simulink model "KF_R_estimation"  (R2021b)
settings: Solver=FixedStepAuto  StartTime=0.0  StopTime=20  MaxStep=1  MinStep=1e-3  RelTol=1e-3
values from neighbouring files (symbols this model uses):
  delta_t = 1/fs    (= 0.001)    [Extended_kalman_filter.m]    (also in kalman_filter.m)
  fs = 1000    [Extended_kalman_filter.m]    (also in kalman_filter.m)
  H = [0,1,1,0,0,0 ... (first row only)    [Extended_kalman_filter.m]    (also in kalman_filter.m = [1,0,1])
  H_2 = [1,0,0,0,1,0 ... (first row only)    [kalman_filter.m]
  I0_off = 20    [kalman_filter.m]
  I_var = I_sig^2    (= 1)    [kalman_filter.m]
  Ids_gain = 10    [kalman_filter.m]
  lamda = 0.95    [Extended_kalman_filter.m]    (also in kalman_filter.m)
  P = P - K*Gm*P    [Extended_kalman_filter.m]    (also in kalman_filter.m = [10,0,0)
  P_3 = [100,0,0,0,0,0 ... (first row only)    [kalman_filter.m]
  Q_2 = [5,0,0,0,0,0 ... (first row only)    [kalman_filter.m]
  Qi = [5,0,0 ... (first row only)    [kalman_filter.m]
  Qv = [5,0,0 ... (first row only)    [kalman_filter.m]
  R_2 = [I_var, 0 ... (first row only)    [kalman_filter.m]
  Ri = I_var    (= 1)    [kalman_filter.m]
  Rv = V_var    (= 1)    [kalman_filter.m]
  V0_off = 0.2    [kalman_filter.m]
  V_var = V_sig^2    (= 1)    [kalman_filter.m]
  Vds_gain = 1    [kalman_filter.m]
  X_kal = X_kal + K*(y_kal(:,k)-ym)    [Extended_kalman_filter.m]    (also in kalman_filter.m = [0;0;0])
  X_kal_2 = [0;0;0;0;1;2]    [kalman_filter.m]
undefined symbols (not defined in the file or in its folder): parameters_a, parameters_b, parameters_c
libraries: simulink x5, ctrlSharedLib x3
settings Model: Creator=Mahmoud  LastModifiedBy=Q540534
settings SolverCC: AlgebraicLoopSolver=LineSearch
settings DebuggingCC: SFMachineParentedDataDiag=warning  ArithmeticOperatorsInVariantConditions=warning
settings SFSimCC: CustomCodeUndefinedFunction=UseInterfaceOnly

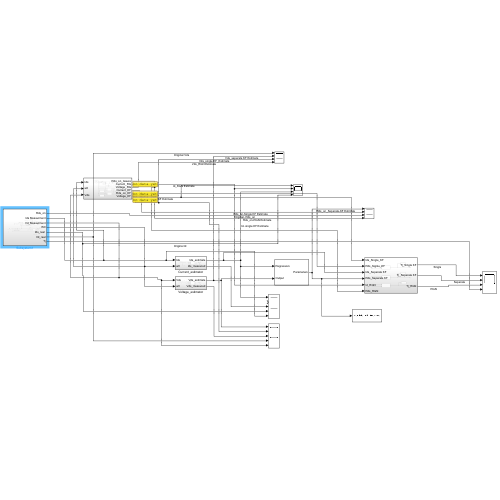
[thumbnail: Simulink's stored preview of the top-level diagram]
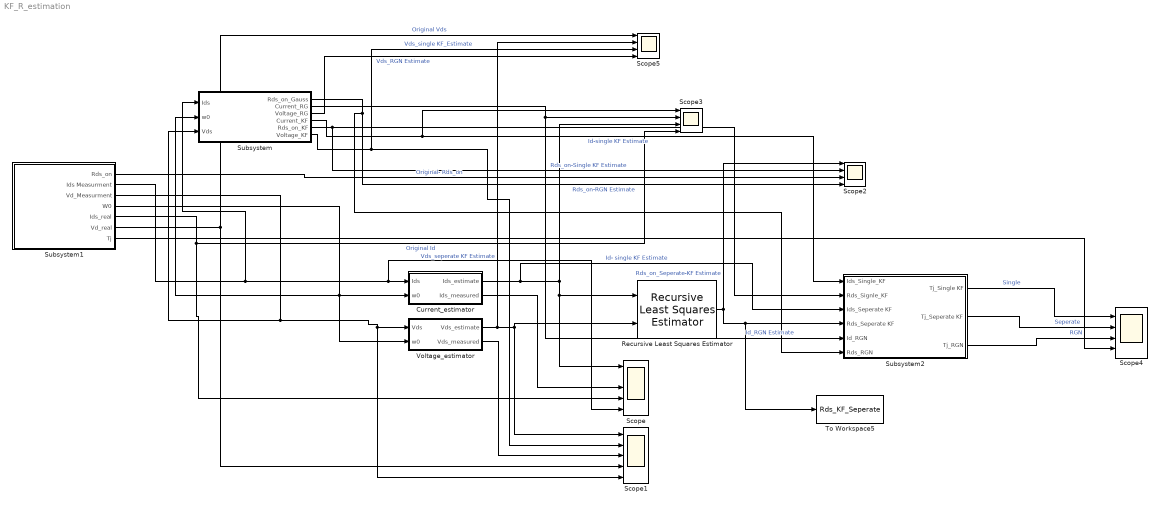
== system KF_R_estimation ==
  Current_estimator : Subsystem
  Recursive Least Squares Estimator : ctrlSharedLib/Recursive Least Squares Estimator  InitialEstimateSource=None  InitialParameterData=1  P0=1  InitialRegressors=0  InitialOutputs=0  History=Finite  WindowLength=50  EstimationMethod=Forgetting Factor  AdaptationParameter=1  HasTimeVaryingAdaptationParameter=off  NormalizationBias=eps  OutputError=off  OutputP=off  AddEnablePort=off  InputProcessing=Sample-based  Ts=delta_t
      settings: SourceProductBaseCode=CT,ID
  Scope : Scope  NumInputPorts=5
  Scope1 : Scope  NumInputPorts=5
  Scope{2..5} (4 alike) : Scope  NumInputPorts=4
  Subsystem : Subsystem
  Subsystem1 : Subsystem
  Subsystem2 : Subsystem
  To Workspace5 : ToWorkspace  VariableName=Rds_KF_Seperate  SaveFormat=Timeseries  SampleTime=-1
  Voltage_estimator : Subsystem
  wires:
  Subsystem1/2(Ids Measurment) -> Scope/5, Current_estimator/1(Ids), Subsystem/1(Ids)
  Current_estimator/1(Ids_estimate) -> Subsystem2/3(Ids_Seperate KF), Scope3/3, Scope/1, Recursive Least Squares Estimator/1  "Id- single KF Estimate"
  Subsystem1/4(W0) -> Current_estimator/2(w0), Subsystem/2(w0), Voltage_estimator/2(w0)
  Subsystem1/3(Vd_Measurment) -> Voltage_estimator/1(Vds), Scope1/5, Subsystem/3(Vds)
  Voltage_estimator/1(Vds_estimate) -> Recursive Least Squares Estimator/2, Scope1/1, Scope5/2  "Vds_seperate KF Estimate"
  Current_estimator/2(Ids_measured) -> Scope/3
  Subsystem1/5("Ids_real ") -> Scope/4, Scope3/4  "Original Id"
  Voltage_estimator/2(Vds_measured) -> Scope1/3
  Subsystem1/6(Vd_real) -> Scope1/4, Scope5/1  "Original Vds"
  Recursive Least Squares Estimator/1 -> Scope2/1, To Workspace5/1, Subsystem2/4(Rds_Seperate KF)  "Rds_on_Seperate-KF Estimate"
  Subsystem1/7(Tj) -> Scope4/4
  Subsystem1/1(Rds_on) -> Scope2/3  "Original- Rds_on"
  Subsystem/1(Rds_on_Gauss) -> Subsystem2/6(Rds_RGN), Scope2/4  "Rds_on-RGN Estimate"
  Subsystem/5(Rds_on_KF) -> Subsystem2/2(Rds_Signle_KF), Scope2/2  "Rds_on-Single KF Estimate"
  Subsystem/4(Current_KF) -> Subsystem2/1(Ids_Single_KF), Scope3/1  "Id-single KF Estimate"
  Subsystem/2(Current_RG) -> Scope3/2, Subsystem2/5(Id_RGN)  "Id_RGN Estimate"
  Subsystem/6(Voltage_KF) -> Scope1/2, Scope5/3  "Vds_single KF_Estimate"
  Subsystem/3(Voltage_RG) -> Scope5/4  "Vds_RGN Estimate"
  Subsystem2/1(Tj_Single KF) -> Scope4/1  "Single"
  Subsystem2/2(Tj_Seperate KF) -> Scope4/2  "Seperate"
  Subsystem2/3(Tj_RGN) -> Scope4/3  "RGN"

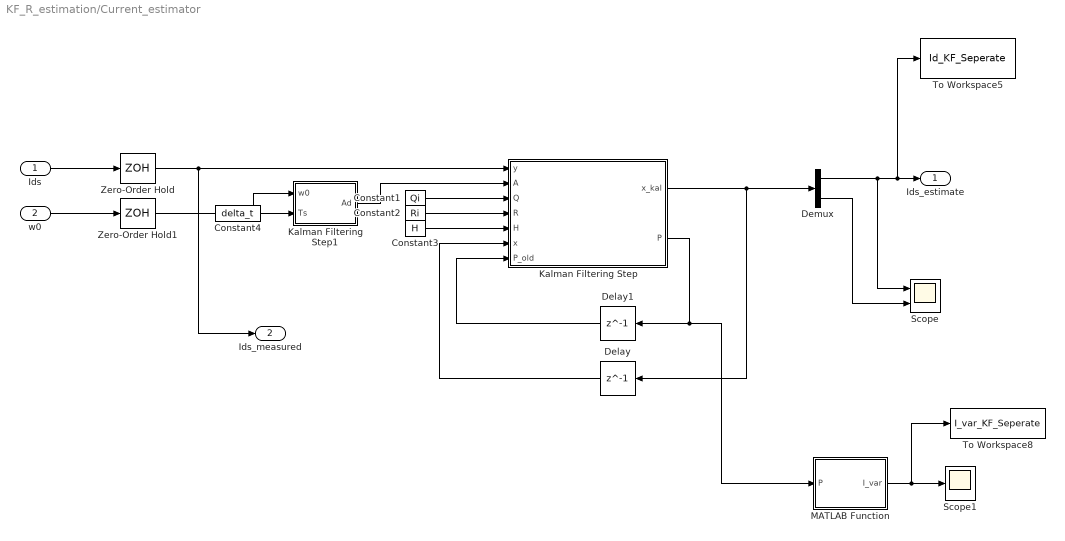
== system KF_R_estimation/Current_estimator ==
  Ids : Inport
  w0 : Inport  Port=2
  Constant1 : Constant  Value=Qi  VectorParams1D=off
  Constant2 : Constant  Value=Ri  VectorParams1D=off
  Constant3 : Constant  Value=H  VectorParams1D=off
  Constant4 : Constant  Value=delta_t  VectorParams1D=off
  Delay : Delay  DelayLength=1  InitialCondition=[0;0;0]  SampleTime=delta_t
  Delay1 : Delay  DelayLength=1  InitialCondition=P  SampleTime=delta_t
  Demux : Demux  Outputs=3
  Kalman Filtering Step : MATLAB Function  TreatAsAtomicUnit=on
  Kalman Filtering Step1 : MATLAB Function  TreatAsAtomicUnit=on
  MATLAB Function : MATLAB Function  TreatAsAtomicUnit=on
  Scope : Scope  NumInputPorts=2
  Scope1 : Scope
  To Workspace5 : ToWorkspace  VariableName=Id_KF_Seperate  SaveFormat=Timeseries  SampleTime=-1
  To Workspace8 : ToWorkspace  VariableName=I_var_KF_Seperate  SaveFormat=Timeseries  SampleTime=-1
  Zero-Order Hold : ZeroOrderHold  SampleTime=delta_t
  Zero-Order Hold1 : ZeroOrderHold  SampleTime=delta_t
  Ids_estimate : Outport  VectorParamsAs1DForOutWhenUnconnected=off
  Ids_measured : Outport  Port=2  VectorParamsAs1DForOutWhenUnconnected=off
  wires:
  Kalman Filtering Step/1(x_kal) -> Demux/1, Delay/1
  Kalman Filtering Step1/1(Ad) -> Kalman Filtering Step/2(A)
  Kalman Filtering Step/2(P) -> MATLAB Function/1(P), Delay1/1
  Delay/1 -> Kalman Filtering Step/6(x)
  Ids/1 -> Zero-Order Hold/1
  Constant1/1 -> Kalman Filtering Step/3(Q)
  Delay1/1 -> Kalman Filtering Step/7(P_old)
  Constant2/1 -> Kalman Filtering Step/4(R)
  Constant3/1 -> Kalman Filtering Step/5(H)
  Demux/1 -> Scope/1, To Workspace5/1, Ids_estimate/1
  Zero-Order Hold/1 -> Ids_measured/1, Kalman Filtering Step/1(y)
  w0/1 -> Zero-Order Hold1/1
  Zero-Order Hold1/1 -> Kalman Filtering Step1/1(w0)
  Constant4/1 -> Kalman Filtering Step1/2(Ts)
  Demux/3 -> Scope/2
  MATLAB Function/1(I_var) -> To Workspace8/1, Scope1/1

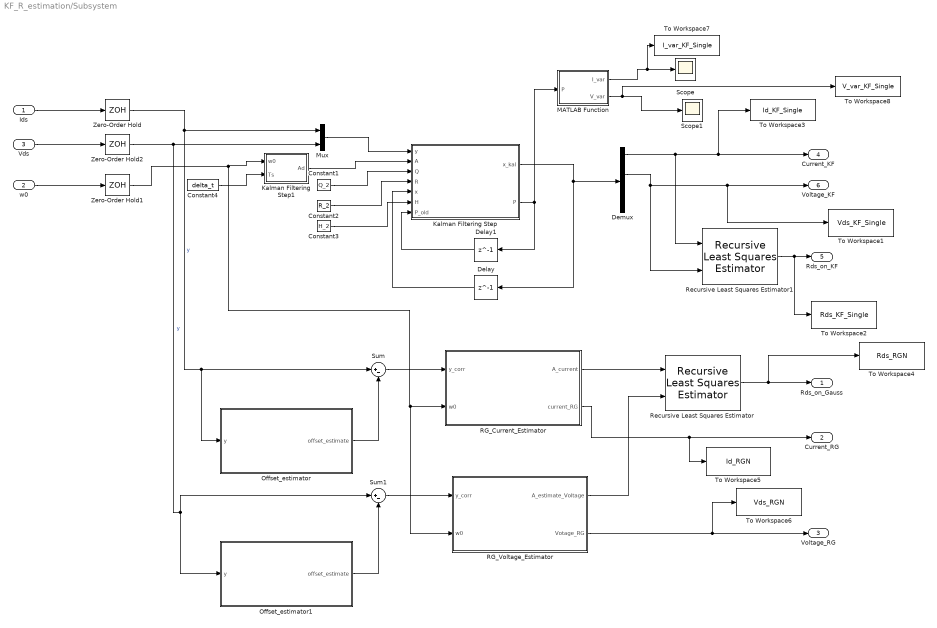
== system KF_R_estimation/Subsystem ==
  Ids : Inport
  w0 : Inport  Port=2
  Vds : Inport  Port=3
  Constant1 : Constant  Value=Q_2  VectorParams1D=off
  Constant2 : Constant  Value=R_2  VectorParams1D=off
  Constant3 : Constant  Value=H_2  VectorParams1D=off
  Constant4 : Constant  Value=delta_t  VectorParams1D=off
  Delay : Delay  DelayLength=1  InitialCondition=X_kal_2  SampleTime=delta_t
  Delay1 : Delay  DelayLength=1  InitialCondition=P_3  SampleTime=delta_t
  Demux : Demux  Outputs=6
  Kalman Filtering Step : MATLAB Function  TreatAsAtomicUnit=on
  Kalman Filtering Step1 : MATLAB Function  TreatAsAtomicUnit=on
  MATLAB Function : MATLAB Function  TreatAsAtomicUnit=on
  Mux : Mux  Inputs=2
  Offset_estimator : Subsystem
  Offset_estimator1 : Subsystem
  RG_Current_Estimator : Subsystem
  RG_Voltage_Estimator : Subsystem
  Recursive Least Squares Estimator : ctrlSharedLib/Recursive Least Squares Estimator  InitialEstimateSource=None  InitialParameterData=1  P0=1  InitialRegressors=0  InitialOutputs=0  History=Finite  WindowLength=25  EstimationMethod=Forgetting Factor  AdaptationParameter=1  HasTimeVaryingAdaptationParameter=off  NormalizationBias=eps  OutputError=off  OutputP=off  AddEnablePort=off  InputProcessing=Sample-based  Ts=delta_t
      settings: SourceProductBaseCode=CT,ID
  Recursive Least Squares Estimator1 : ctrlSharedLib/Recursive Least Squares Estimator  InitialEstimateSource=None  InitialParameterData=1  P0=1  InitialRegressors=0  InitialOutputs=0  History=Finite  WindowLength=50  EstimationMethod=Forgetting Factor  AdaptationParameter=1  HasTimeVaryingAdaptationParameter=off  NormalizationBias=eps  OutputError=off  OutputP=off  AddEnablePort=off  InputProcessing=Sample-based  Ts=delta_t
      settings: SourceProductBaseCode=CT,ID
  Scope : Scope
  Scope1 : Scope
  Sum : Sum  Inputs=|+-
  Sum1 : Sum  Inputs=|+-
  To Workspace1 : ToWorkspace  VariableName=Vds_KF_Single  SaveFormat=Timeseries  SampleTime=-1
  To Workspace2 : ToWorkspace  VariableName=Rds_KF_Single  SaveFormat=Timeseries  SampleTime=-1
  To Workspace3 : ToWorkspace  VariableName=Id_KF_Single  SaveFormat=Timeseries  SampleTime=-1
  To Workspace4 : ToWorkspace  VariableName=Rds_RGN  SaveFormat=Timeseries  SampleTime=-1
  To Workspace5 : ToWorkspace  VariableName=Id_RGN  SaveFormat=Timeseries  SampleTime=-1
  To Workspace6 : ToWorkspace  VariableName=Vds_RGN  SaveFormat=Timeseries  SampleTime=-1
  To Workspace7 : ToWorkspace  VariableName=I_var_KF_Single  SaveFormat=Timeseries  SampleTime=-1
  To Workspace8 : ToWorkspace  VariableName=V_var_KF_Single  SaveFormat=Timeseries  SampleTime=-1
  Zero-Order Hold : ZeroOrderHold  SampleTime=delta_t
  Zero-Order Hold1 : ZeroOrderHold  SampleTime=delta_t
  Zero-Order Hold2 : ZeroOrderHold  SampleTime=delta_t
  Rds_on_Gauss : Outport  VectorParamsAs1DForOutWhenUnconnected=off
  Current_RG : Outport  Port=2  VectorParamsAs1DForOutWhenUnconnected=off
  Voltage_RG : Outport  Port=3  VectorParamsAs1DForOutWhenUnconnected=off
  Current_KF : Outport  Port=4  VectorParamsAs1DForOutWhenUnconnected=off
  Rds_on_KF : Outport  Port=5  VectorParamsAs1DForOutWhenUnconnected=off
  Voltage_KF : Outport  Port=6  VectorParamsAs1DForOutWhenUnconnected=off
  wires:
  Constant2/1 -> Kalman Filtering Step/4(R)
  Zero-Order Hold1/1 -> Kalman Filtering Step1/1(w0), RG_Voltage_Estimator/2(w0), RG_Current_Estimator/2(w0)
  Constant4/1 -> Kalman Filtering Step1/2(Ts)
  w0/1 -> Zero-Order Hold1/1
  Kalman Filtering Step/1(x_kal) -> Demux/1, Delay/1
  Delay/1 -> Kalman Filtering Step/5(x)
  Kalman Filtering Step/2(P) -> Delay1/1, MATLAB Function/1(P)
  Delay1/1 -> Kalman Filtering Step/7(P_old)
  Ids/1 -> Zero-Order Hold/1
  Kalman Filtering Step1/1(Ad) -> Kalman Filtering Step/2(A)
  Constant1/1 -> Kalman Filtering Step/3(Q)
  Vds/1 -> Zero-Order Hold2/1
  Mux/1 -> Kalman Filtering Step/1(y)
  Offset_estimator/1(offset_estimate) -> Sum/2
  Zero-Order Hold/1 -> Mux/1, Offset_estimator/1(y), Sum/1  "y"
  RG_Current_Estimator/1(A_current) -> Recursive Least Squares Estimator/1
  Sum/1 -> RG_Current_Estimator/1(y_corr)
  Zero-Order Hold2/1 -> Mux/2, Offset_estimator1/1(y), Sum1/1  "y"
  Offset_estimator1/1(offset_estimate) -> Sum1/2
  Sum1/1 -> RG_Voltage_Estimator/1(y_corr)
  RG_Voltage_Estimator/1(A_estimate_Voltage) -> Recursive Least Squares Estimator/2
  Recursive Least Squares Estimator/1 -> To Workspace4/1, Rds_on_Gauss/1
  RG_Current_Estimator/2(current_RG) -> To Workspace5/1, Current_RG/1
  RG_Voltage_Estimator/2(Votage_RG) -> To Workspace6/1, Voltage_RG/1
  Demux/1 -> To Workspace3/1, Current_KF/1, Recursive Least Squares Estimator1/1
  Recursive Least Squares Estimator1/1 -> To Workspace2/1, Rds_on_KF/1
  Constant3/1 -> Kalman Filtering Step/6(H)
  Demux/3 -> Recursive Least Squares Estimator1/2, To Workspace1/1, Voltage_KF/1
  MATLAB Function/1(I_var) -> To Workspace7/1, Scope/1
  MATLAB Function/2(V_var) -> Scope1/1, To Workspace8/1

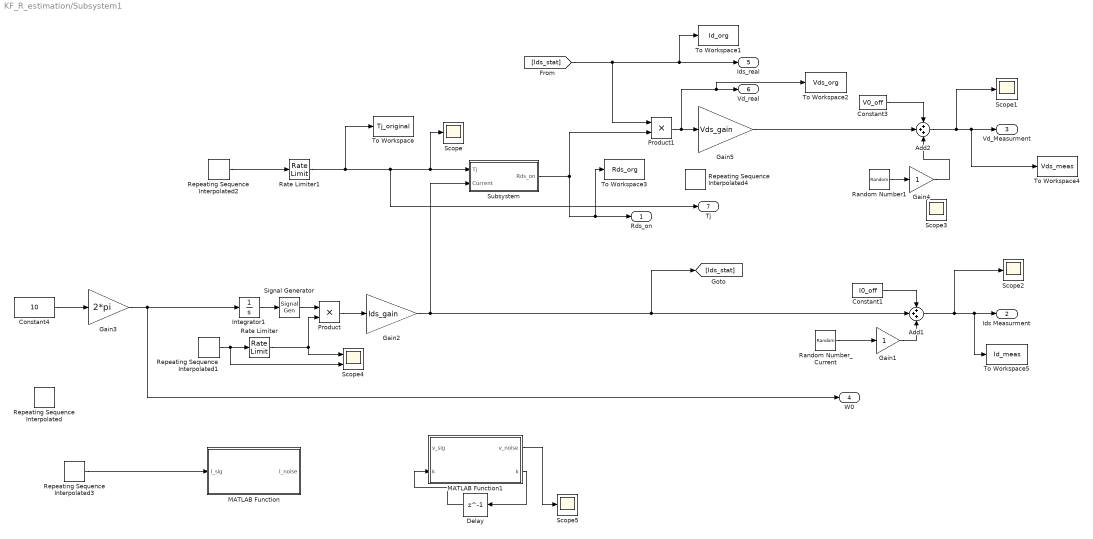
== system KF_R_estimation/Subsystem1 ==
  Add1 : Sum  Inputs=+++
  Add2 : Sum  Inputs=+++
  Constant1 : Constant  Value=I0_off
  Constant3 : Constant  Value=V0_off
  Constant4 : Constant  Value=10
  Delay : Delay  DelayLength=1  InitialCondition=0
  Gain1 : Gain
  Gain2 : Gain  Gain=Ids_gain
  Gain3 : Gain  Gain=2*pi
  Gain4 : Gain
  Gain5 : Gain  Gain=Vds_gain
  Integrator1 : Integrator
  MATLAB Function : MATLAB Function  TreatAsAtomicUnit=on
  MATLAB Function1 : MATLAB Function  TreatAsAtomicUnit=on
  Product : Product
  Product1 : Product
  Random Number1 : RandomNumber  Variance=V_var  SampleTime=delta_t
  Random Number_Current : RandomNumber  Variance=I_var  SampleTime=delta_t
  Rate Limiter : RateLimiter  RisingSlewLimit=2  FallingSlewLimit=-2  InitialCondition=3
  Rate Limiter1 : RateLimiter  RisingSlewLimit=200  FallingSlewLimit=-200  InitialCondition=3
  Repeating Sequence Interpolated : simulink/Sources/Repeating Sequence Interpolated  OutValues=5*[3 1 4 2 1].'  TimeValues=10*[0 0.1 0.5 0.6 1].'  LookUpMeth=Interpolation-Use End Values  tsamp=-1  OutMin=[]  OutMax=[]  OutDataTypeStr=double  OutputDataTypeScalingMode=double  OutDataType=fixdt(0,8)  OutScaling=2^-10
  Repeating Sequence Interpolated1 : simulink/Sources/Repeating Sequence Interpolated  OutValues=[3 3 5 5 2 2]  TimeValues=10*[0 0.2 0.4 0.6 0.8 1]  LookUpMeth=Interpolation-Use End Values  tsamp=-1  OutMin=[]  OutMax=[]  OutDataTypeStr=double  OutputDataTypeScalingMode=double  OutDataType=fixdt(0,8)  OutScaling=2^-10
  Repeating Sequence Interpolated2 : simulink/Sources/Repeating Sequence Interpolated  OutValues=[60 150 100 200 100 200]  TimeValues=10*[0 0.2 0.4 0.6 0.8 1]  LookUpMeth=Interpolation-Use End Values  tsamp=-1  OutMin=[]  OutMax=[]  OutDataTypeStr=double  OutputDataTypeScalingMode=double  OutDataType=fixdt(0,8)  OutScaling=2^-10
  Repeating Sequence Interpolated3 : simulink/Sources/Repeating Sequence Interpolated  OutValues=[5 10 15 20 30 50]  TimeValues=10*[0 0.2 0.4 0.6 0.8 1]  LookUpMeth=Interpolation-Use End Values  tsamp=delta_t  OutMin=[]  OutMax=[]  OutDataTypeStr=double  OutputDataTypeScalingMode=double  OutDataType=fixdt(0,8)  OutScaling=2^-10
  Repeating Sequence Interpolated4 : simulink/Sources/Repeating Sequence Interpolated  OutValues=[10 5 20 40 50 35]  TimeValues=10*[0 0.2 0.4 0.6 0.8 1]  LookUpMeth=Interpolation-Use End Values  tsamp=-1  OutMin=[]  OutMax=[]  OutDataTypeStr=double  OutputDataTypeScalingMode=double  OutDataType=fixdt(0,8)  OutScaling=2^-10
  Scope{,1..3,5} (5 alike) : Scope
  Scope4 : Scope  NumInputPorts=2
  Signal Generator : SignalGenerator  TimeSource=Use external signal  Units=rad/sec
  Subsystem : Subsystem
  To Workspace : ToWorkspace  VariableName=Tj_original  SaveFormat=Timeseries  SampleTime=-1
  To Workspace1 : ToWorkspace  VariableName=Id_org  SaveFormat=Timeseries  SampleTime=-1
  To Workspace2 : ToWorkspace  VariableName=Vds_org  SaveFormat=Timeseries  SampleTime=-1
  To Workspace3 : ToWorkspace  VariableName=Rds_org  SaveFormat=Timeseries  SampleTime=-1
  To Workspace4 : ToWorkspace  VariableName=Vds_meas  SaveFormat=Timeseries  SampleTime=-1
  To Workspace5 : ToWorkspace  VariableName=Id_meas  SaveFormat=Timeseries  SampleTime=-1
  Rds_on : Outport  VectorParamsAs1DForOutWhenUnconnected=off
  Ids Measurment : Outport  Port=2  VectorParamsAs1DForOutWhenUnconnected=off
  Vd_Measurment : Outport  Port=3  VectorParamsAs1DForOutWhenUnconnected=off
  W0 : Outport  Port=4  VectorParamsAs1DForOutWhenUnconnected=off
  "Ids_real " : Outport  Port=5  VectorParamsAs1DForOutWhenUnconnected=off
  Vd_real : Outport  Port=6  VectorParamsAs1DForOutWhenUnconnected=off
  Tj : Outport  Port=7  VectorParamsAs1DForOutWhenUnconnected=off
  wires:
  Constant1/1 -> Add1/1
  Product/1 -> Gain2/1
  Add1/1 -> Scope2/1, To Workspace5/1, Ids Measurment/1
  Integrator1/1 -> Signal Generator/1
  Gain2/1 -> [Ids_stat], Add1/2, Subsystem/2(Current)
  Signal Generator/1 -> Product/1
  Gain1/1 -> Add1/3
  Gain3/1 -> W0/1, Integrator1/1
  Repeating Sequence Interpolated1/1 -> Scope4/2, Rate Limiter/1
  Repeating Sequence Interpolated2/1 -> Rate Limiter1/1
  Add2/1 -> Scope1/1, To Workspace4/1, Vd_Measurment/1
  Constant3/1 -> Add2/1
  Gain4/1 -> Add2/3
  Constant4/1 -> Gain3/1
  Gain5/1 -> Add2/2
  Rate Limiter/1 -> Product/2, Scope4/1
  Subsystem/1(Rds_on) -> Product1/2, To Workspace3/1, Rds_on/1
  [Ids_stat] -> Product1/1, To Workspace1/1, "Ids_real "/1
  Rate Limiter1/1 -> To Workspace/1, Tj/1, Scope/1, Subsystem/1(Tj)
  Product1/1 -> Gain5/1, To Workspace2/1, Vd_real/1
  Repeating Sequence Interpolated3/1 -> MATLAB Function/1(I_sig)
  Delay/1 -> MATLAB Function1/2("k ")
  MATLAB Function1/2(k) -> Delay/1
  Random Number_Current/1 -> Gain1/1
  Random Number1/1 -> Gain4/1
  MATLAB Function1/1(v_noise) -> Scope5/1

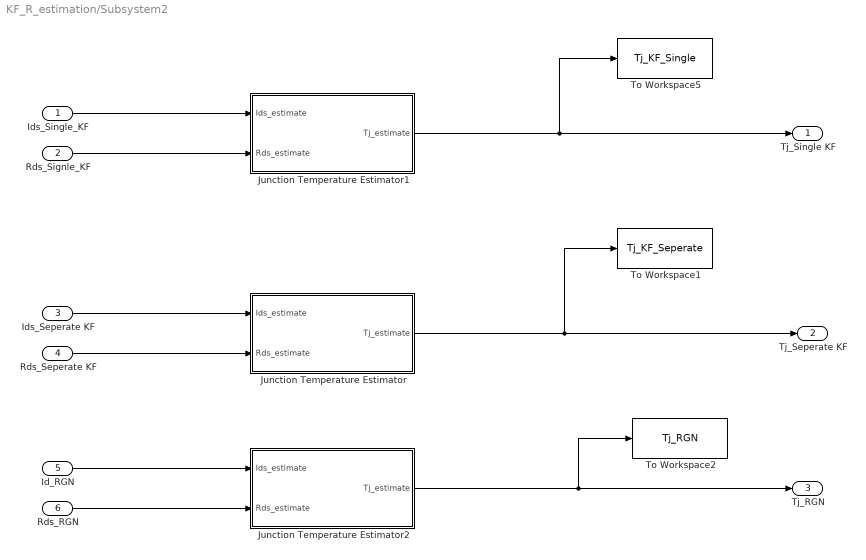
== system KF_R_estimation/Subsystem2 ==
  Ids_Single_KF : Inport
  Rds_Signle_KF : Inport  Port=2
  Ids_Seperate KF : Inport  Port=3
  Rds_Seperate KF : Inport  Port=4
  Id_RGN : Inport  Port=5
  Rds_RGN : Inport  Port=6
  Junction Temperature Estimator : Subsystem
  Junction Temperature Estimator1 : Subsystem
  Junction Temperature Estimator2 : Subsystem
  To Workspace1 : ToWorkspace  VariableName=Tj_KF_Seperate  SaveFormat=Timeseries  SampleTime=-1
  To Workspace2 : ToWorkspace  VariableName=Tj_RGN  SaveFormat=Timeseries  SampleTime=-1
  To Workspace5 : ToWorkspace  VariableName=Tj_KF_Single  SaveFormat=Timeseries  SampleTime=-1
  Tj_Single KF : Outport
  Tj_Seperate KF : Outport  Port=2
  Tj_RGN : Outport  Port=3
  wires:
  Junction Temperature Estimator1/1(Tj_estimate) -> To Workspace5/1, Tj_Single KF/1
  Junction Temperature Estimator/1(Tj_estimate) -> To Workspace1/1, Tj_Seperate KF/1
  Junction Temperature Estimator2/1(Tj_estimate) -> To Workspace2/1, Tj_RGN/1
  Ids_Single_KF/1 -> Junction Temperature Estimator1/1(Ids_estimate)
  Rds_Signle_KF/1 -> Junction Temperature Estimator1/2(Rds_estimate)
  Ids_Seperate KF/1 -> Junction Temperature Estimator/1(Ids_estimate)
  Rds_Seperate KF/1 -> Junction Temperature Estimator/2(Rds_estimate)
  Id_RGN/1 -> Junction Temperature Estimator2/1(Ids_estimate)
  Rds_RGN/1 -> Junction Temperature Estimator2/2(Rds_estimate)

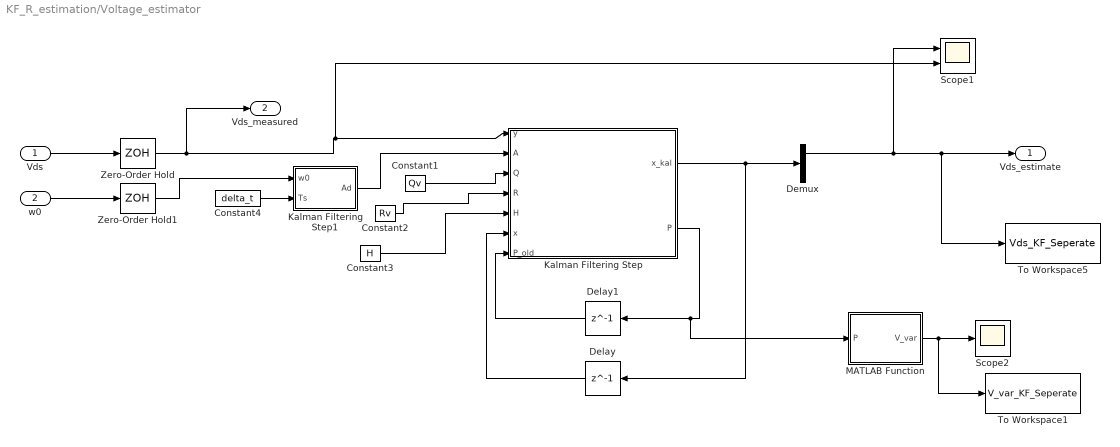
== system KF_R_estimation/Voltage_estimator ==
  Vds : Inport
  w0 : Inport  Port=2
  Constant1 : Constant  Value=Qv  VectorParams1D=off
  Constant2 : Constant  Value=Rv  VectorParams1D=off
  Constant3 : Constant  Value=H  VectorParams1D=off
  Constant4 : Constant  Value=delta_t  VectorParams1D=off
  Delay : Delay  DelayLength=1  InitialCondition=X_kal  SampleTime=delta_t
  Delay1 : Delay  DelayLength=1  InitialCondition=P  SampleTime=delta_t
  Demux : Demux  Outputs=3
  Kalman Filtering Step : MATLAB Function  TreatAsAtomicUnit=on
  Kalman Filtering Step1 : MATLAB Function  TreatAsAtomicUnit=on
  MATLAB Function : MATLAB Function  TreatAsAtomicUnit=on
  Scope1 : Scope  NumInputPorts=2
  Scope2 : Scope
  To Workspace1 : ToWorkspace  VariableName=V_var_KF_Seperate  SaveFormat=Timeseries  SampleTime=-1
  To Workspace5 : ToWorkspace  VariableName=Vds_KF_Seperate  SaveFormat=Timeseries  SampleTime=-1
  Zero-Order Hold : ZeroOrderHold  SampleTime=delta_t
  Zero-Order Hold1 : ZeroOrderHold  SampleTime=delta_t
  Vds_estimate : Outport  VectorParamsAs1DForOutWhenUnconnected=off
  Vds_measured : Outport  Port=2  VectorParamsAs1DForOutWhenUnconnected=off
  wires:
  Constant4/1 -> Kalman Filtering Step1/2(Ts)
  Zero-Order Hold1/1 -> Kalman Filtering Step1/1(w0)
  w0/1 -> Zero-Order Hold1/1
  Zero-Order Hold/1 -> Vds_measured/1, Scope1/2, Kalman Filtering Step/1(y)
  Constant2/1 -> Kalman Filtering Step/4(R)
  Delay1/1 -> Kalman Filtering Step/7(P_old)
  Constant1/1 -> Kalman Filtering Step/3(Q)
  Vds/1 -> Zero-Order Hold/1
  Delay/1 -> Kalman Filtering Step/6(x)
  Kalman Filtering Step/2(P) -> MATLAB Function/1(P), Delay1/1
  Kalman Filtering Step1/1(Ad) -> Kalman Filtering Step/2(A)
  Constant3/1 -> Kalman Filtering Step/5(H)
  MATLAB Function/1(V_var) -> To Workspace1/1, Scope2/1
  Kalman Filtering Step/1(x_kal) -> Demux/1, Delay/1
  Demux/1 -> Scope1/1, To Workspace5/1, Vds_estimate/1

== system KF_R_estimation/Subsystem/Offset_estimator ==
  y : Inport
  Delay2 : Delay  DelayLength=1  InitialCondition=0
  Delay3 : Delay  DelayLength=1  InitialCondition=0
  MATLAB Function : MATLAB Function  TreatAsAtomicUnit=on
  offset_estimate : Outport  VectorParamsAs1DForOutWhenUnconnected=off
  wires:
  MATLAB Function/2(k_2) -> Delay3/1
  Delay2/1 -> MATLAB Function/1(offset_before)
  Delay3/1 -> MATLAB Function/3("k_2 ")
  MATLAB Function/1(offset_after) -> offset_estimate/1, Delay2/1
  y/1 -> MATLAB Function/2(y)

== system KF_R_estimation/Subsystem/Offset_estimator1 ==
  y : Inport
  Delay2 : Delay  DelayLength=1  InitialCondition=0
  Delay3 : Delay  DelayLength=1  InitialCondition=0
  MATLAB Function : MATLAB Function  TreatAsAtomicUnit=on
  offset_estimate : Outport  VectorParamsAs1DForOutWhenUnconnected=off
  wires:
  MATLAB Function/2(k_2) -> Delay3/1
  Delay2/1 -> MATLAB Function/1(offset_before)
  Delay3/1 -> MATLAB Function/3("k_2 ")
  MATLAB Function/1(offset_after) -> offset_estimate/1, Delay2/1
  y/1 -> MATLAB Function/2(y)

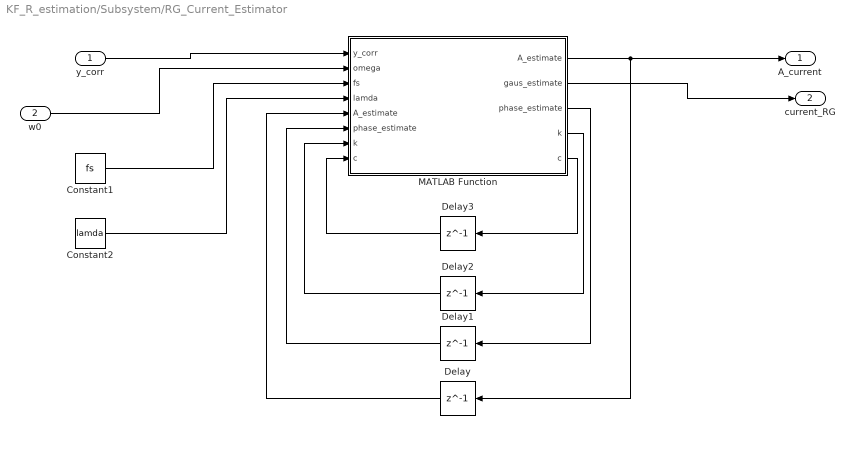
== system KF_R_estimation/Subsystem/RG_Current_Estimator ==
  y_corr : Inport
  w0 : Inport  Port=2
  Constant1 : Constant  Value=fs
  Constant2 : Constant  Value=lamda
  Delay : Delay  DelayLength=1  InitialCondition=1
  Delay1 : Delay  DelayLength=1  InitialCondition=0
  Delay2 : Delay  DelayLength=1  InitialCondition=0
  Delay3 : Delay  DelayLength=1  InitialCondition=0
  MATLAB Function : MATLAB Function  TreatAsAtomicUnit=on
  A_current : Outport  VectorParamsAs1DForOutWhenUnconnected=off
  current_RG : Outport  Port=2  VectorParamsAs1DForOutWhenUnconnected=off
  wires:
  MATLAB Function/1(A_estimate) -> Delay/1, A_current/1
  MATLAB Function/3(phase_estimate) -> Delay1/1
  y_corr/1 -> MATLAB Function/1(y_corr)
  w0/1 -> MATLAB Function/2(omega)
  Constant1/1 -> MATLAB Function/3(fs)
  Delay1/1 -> MATLAB Function/6("phase_estimate ")
  Delay/1 -> MATLAB Function/5("A_estimate ")
  MATLAB Function/4(k) -> Delay2/1
  Delay2/1 -> MATLAB Function/7("k ")
  MATLAB Function/5(c) -> Delay3/1
  Constant2/1 -> MATLAB Function/4(lamda)
  Delay3/1 -> MATLAB Function/8("c ")
  MATLAB Function/2(gaus_estimate) -> current_RG/1

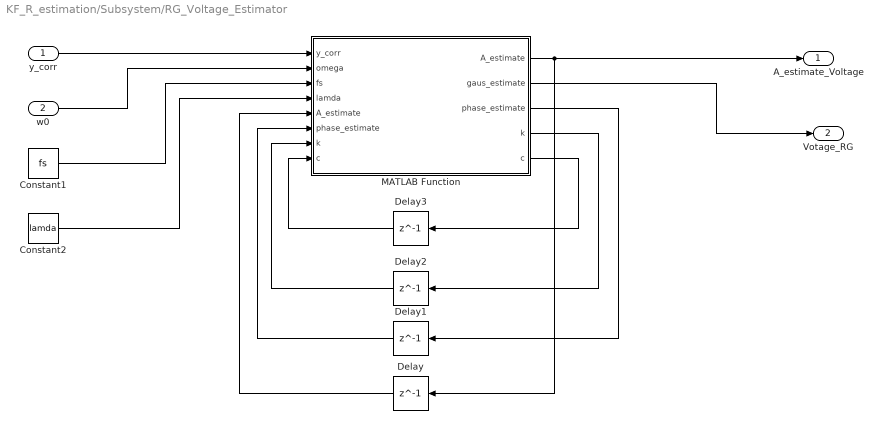
== system KF_R_estimation/Subsystem/RG_Voltage_Estimator ==
  y_corr : Inport
  w0 : Inport  Port=2
  Constant1 : Constant  Value=fs
  Constant2 : Constant  Value=lamda
  Delay : Delay  DelayLength=1  InitialCondition=1
  Delay1 : Delay  DelayLength=1  InitialCondition=0
  Delay2 : Delay  DelayLength=1  InitialCondition=0
  Delay3 : Delay  DelayLength=1  InitialCondition=0
  MATLAB Function : MATLAB Function  TreatAsAtomicUnit=on
  A_estimate_Voltage : Outport  VectorParamsAs1DForOutWhenUnconnected=off
  Votage_RG : Outport  Port=2  VectorParamsAs1DForOutWhenUnconnected=off
  wires:
  MATLAB Function/1(A_estimate) -> Delay/1, A_estimate_Voltage/1
  MATLAB Function/3(phase_estimate) -> Delay1/1
  y_corr/1 -> MATLAB Function/1(y_corr)
  w0/1 -> MATLAB Function/2(omega)
  Constant1/1 -> MATLAB Function/3(fs)
  Delay1/1 -> MATLAB Function/6("phase_estimate ")
  Delay/1 -> MATLAB Function/5("A_estimate ")
  MATLAB Function/4(k) -> Delay2/1
  Delay2/1 -> MATLAB Function/7("k ")
  MATLAB Function/5(c) -> Delay3/1
  Constant2/1 -> MATLAB Function/4(lamda)
  Delay3/1 -> MATLAB Function/8("c ")
  MATLAB Function/2(gaus_estimate) -> Votage_RG/1

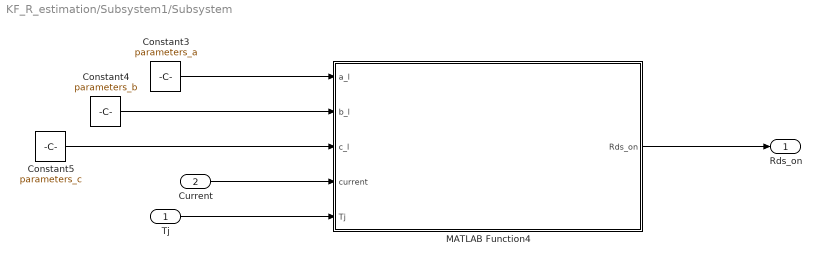
== system KF_R_estimation/Subsystem1/Subsystem ==
  Tj : Inport
  Current : Inport  Port=2
  Constant3 : Constant  Value=parameters_a  VectorParams1D=off
  Constant4 : Constant  Value=parameters_b  VectorParams1D=off
  Constant5 : Constant  Value=parameters_c  VectorParams1D=off
  MATLAB Function4 : MATLAB Function  TreatAsAtomicUnit=on
  Rds_on : Outport  VectorParamsAs1DForOutWhenUnconnected=off
  wires:
  Tj/1 -> MATLAB Function4/5(Tj)
  MATLAB Function4/1(Rds_on) -> Rds_on/1
  Constant3/1 -> MATLAB Function4/1(a_l)
  Constant4/1 -> MATLAB Function4/2(b_l)
  Constant5/1 -> MATLAB Function4/3(c_l)
  Current/1 -> MATLAB Function4/4(current)

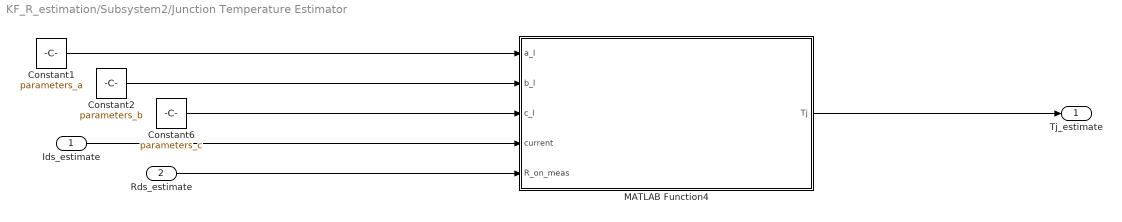
== system KF_R_estimation/Subsystem2/Junction Temperature Estimator ==
  Ids_estimate : Inport
  Rds_estimate : Inport  Port=2
  Constant1 : Constant  Value=parameters_a  VectorParams1D=off
  Constant2 : Constant  Value=parameters_b  VectorParams1D=off
  Constant6 : Constant  Value=parameters_c  VectorParams1D=off
  MATLAB Function4 : MATLAB Function  TreatAsAtomicUnit=on
  Tj_estimate : Outport  VectorParamsAs1DForOutWhenUnconnected=off
  wires:
  Constant2/1 -> MATLAB Function4/2(b_l)
  Ids_estimate/1 -> MATLAB Function4/4(current)
  MATLAB Function4/1(Tj) -> Tj_estimate/1
  Rds_estimate/1 -> MATLAB Function4/5(R_on_meas)
  Constant6/1 -> MATLAB Function4/3(c_l)
  Constant1/1 -> MATLAB Function4/1(a_l)

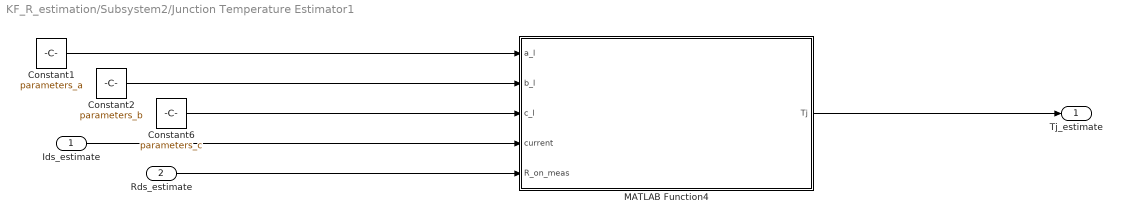
== system KF_R_estimation/Subsystem2/Junction Temperature Estimator1 ==
  Ids_estimate : Inport
  Rds_estimate : Inport  Port=2
  Constant1 : Constant  Value=parameters_a  VectorParams1D=off
  Constant2 : Constant  Value=parameters_b  VectorParams1D=off
  Constant6 : Constant  Value=parameters_c  VectorParams1D=off
  MATLAB Function4 : MATLAB Function  TreatAsAtomicUnit=on
  Tj_estimate : Outport  VectorParamsAs1DForOutWhenUnconnected=off
  wires:
  Constant2/1 -> MATLAB Function4/2(b_l)
  Ids_estimate/1 -> MATLAB Function4/4(current)
  MATLAB Function4/1(Tj) -> Tj_estimate/1
  Rds_estimate/1 -> MATLAB Function4/5(R_on_meas)
  Constant6/1 -> MATLAB Function4/3(c_l)
  Constant1/1 -> MATLAB Function4/1(a_l)

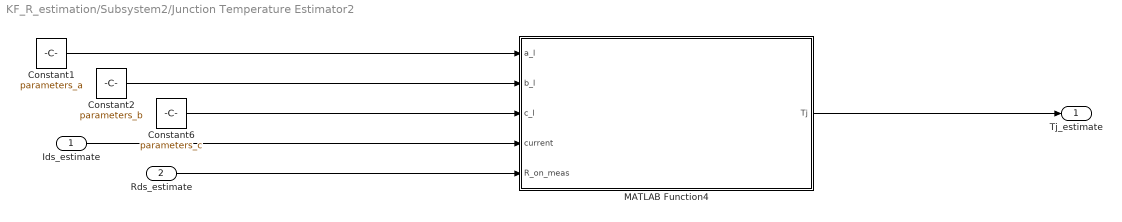
== system KF_R_estimation/Subsystem2/Junction Temperature Estimator2 ==
  Ids_estimate : Inport
  Rds_estimate : Inport  Port=2
  Constant1 : Constant  Value=parameters_a  VectorParams1D=off
  Constant2 : Constant  Value=parameters_b  VectorParams1D=off
  Constant6 : Constant  Value=parameters_c  VectorParams1D=off
  MATLAB Function4 : MATLAB Function  TreatAsAtomicUnit=on
  Tj_estimate : Outport  VectorParamsAs1DForOutWhenUnconnected=off
  wires:
  Constant2/1 -> MATLAB Function4/2(b_l)
  Ids_estimate/1 -> MATLAB Function4/4(current)
  MATLAB Function4/1(Tj) -> Tj_estimate/1
  Rds_estimate/1 -> MATLAB Function4/5(R_on_meas)
  Constant6/1 -> MATLAB Function4/3(c_l)
  Constant1/1 -> MATLAB Function4/1(a_l)

== matlab function KF_R_estimation/Subsystem2/Junction Temperature Estimator/MATLAB Function4 ==
  data: a_l input; b_l input; c_l input; Tj output; current input; R_on_meas input
function Tj = estimate_Tj(a_l,b_l,c_l,current,R_on_meas)
     I=[1; current; current^2; current^3;current^4;current.^5;current.^6]
     a=  a_l*I*1000 
     b=  b_l*I*1000
     c=  c_l*I*1000
     root_part=sqrt(abs(b^2-4*c*(a-R_on_meas))); 
     Tj=(-b+root_part)/(2*c) ;
        
end

== matlab function KF_R_estimation/Subsystem/RG_Current_Estimator/MATLAB Function ==
  data: y_corr input; omega input; fs input; lamda input; A_estimate input; phase_estimate input; k input; A_estimate output; gaus_estimate output; phase_estimate output; k output; c output; c input
function [A_estimate,gaus_estimate,phase_estimate,k,c] = fcn(y_corr,omega,fs,lamda,A_estimate,phase_estimate,k,c)
gaus_estimate =0;
c=lamda*c+0.5;
 e=y_corr-A_estimate*sin((omega/fs)*k+phase_estimate);
 phase_estimate_prev=phase_estimate;
 phase_estimate=phase_estimate+cos((omega/fs)*k+phase_estimate)*(e/(A_estimate*c));
 A_estimate=A_estimate+sin((omega/fs)*k+phase_estimate_prev)*(e/c);
 gaus_estimate=A_estimate*sin((omega/fs)*k+phase_estimate);
 k=k+1

== matlab function KF_R_estimation/Subsystem/RG_Voltage_Estimator/MATLAB Function ==
  data: A_estimate output; gaus_estimate output; y_corr input; omega input; fs input; lamda input; A_estimate input; phase_estimate input; k input; phase_estimate output; k output; c output; c input
function [A_estimate,gaus_estimate,phase_estimate,k,c] = fcn(y_corr,omega,fs,lamda,A_estimate,phase_estimate,k,c)
 gaus_estimate=0;
 c=lamda*c+0.5;
 e=y_corr-A_estimate*sin((omega/fs)*k+phase_estimate);
 phase_estimate_prev=phase_estimate;
 phase_estimate=phase_estimate+cos((omega/fs)*k+phase_estimate)*(e/(A_estimate*c));
 A_estimate=A_estimate+sin((omega/fs)*k+phase_estimate_prev)*(e/c);
 gaus_estimate=A_estimate*sin((omega/fs)*k+phase_estimate);
 k=k+1

== matlab function KF_R_estimation/Subsystem/Offset_estimator1/MATLAB Function ==
  data: offset_before input; offset_after output; y input; k_2 input; k_2 output
function [offset_after,k_2] = offset_estimator(offset_before,y, k_2)

offset_after=(offset_before*(k_2)+y)/(k_2+1)
k_2=k_2+1

== matlab function KF_R_estimation/Subsystem2/Junction Temperature Estimator1/MATLAB Function4 ==
  data: a_l input; b_l input; c_l input; Tj output; current input; R_on_meas input
function Tj = estimate_Tj(a_l,b_l,c_l,current,R_on_meas)
     I=[1; current; current^2; current^3;current^4;current.^5;current.^6]
     a=  a_l*I*1000 
     b=  b_l*I*1000
     c=  c_l*I*1000
     root_part=sqrt(abs(b^2-4*c*(a-R_on_meas))); 
     Tj=(-b+root_part)/(2*c) ;
        
end

== matlab function KF_R_estimation/Subsystem2/Junction Temperature Estimator2/MATLAB Function4 ==
  data: a_l input; b_l input; c_l input; Tj output; current input; R_on_meas input
function Tj = estimate_Tj(a_l,b_l,c_l,current,R_on_meas)
     I=[1; current; current^2; current^3;current^4;current.^5;current.^6]
     a=  a_l*I*1000 
     b=  b_l*I*1000
     c=  c_l*I*1000
     root_part=sqrt(abs(b^2-4*c*(a-R_on_meas))); 
     Tj=(-b+root_part)/(2*c) ;
        
end

== matlab function KF_R_estimation/Subsystem1/MATLAB Function ==
  data: I_sig input; I_noise output
function I_noise = fcn(I_sig)
I_noise=randn*I_sig

== matlab function KF_R_estimation/Subsystem1/MATLAB Function1 ==
  data: v_sig input; v_noise output; k input; k output
function [v_noise,k] = random_number_generator(v_sig,k)
rng(k);
v_noise=randn*v_sig
k=k+1

== matlab function KF_R_estimation/Current_estimator/Kalman Filtering Step1 ==
  data: w0 input; Ad output; Ts input
function Ad = A_d(w0,Ts)
Ad =[cos(w0*Ts),sin(w0*Ts)/w0, 0;
    -sin(w0*Ts)*w0,cos(w0*Ts),0;
    0,0,1];

== matlab function KF_R_estimation/Subsystem/MATLAB Function ==
  data: P input; I_var output; V_var output
function [I_var, V_var] = fcn(P)

I_var = P(1,1);
V_var= P(3,3);

== matlab function KF_R_estimation/Current_estimator/MATLAB Function ==
  data: P input; I_var output
function I_var  = fcn(P)

I_var = P(1,1);

== matlab function KF_R_estimation/Voltage_estimator/MATLAB Function ==
  data: P input; V_var output
function V_var  = fcn(P)

V_var = P(1,1);

== matlab function KF_R_estimation/Voltage_estimator/Kalman Filtering Step ==
  data: y input; A input; Q input; R input; H input; x input; x_kal output; P_old input; P output
function [x_kal,P] = kalman_filter(y,A,Q,R,H,x,P_old)
     x_kal = A*x ;
     P = A*P_old*A' + Q;
     ym = H*x_kal;
     Pm = H*P*H' +R;
     K = P*H'*inv(Pm);       
     x_kal = x_kal + K*(y-ym);
     P = P - K*H*P;

== matlab function KF_R_estimation/Current_estimator/Kalman Filtering Step ==
  data: y input; A input; Q input; R input; H input; x input; x_kal output; P_old input; P output
function [x_kal,P] = kalman_filter(y,A,Q,R,H,x,P_old)
     x_kal = A*x ;
     P = A*P_old*A' + Q;

     ym = H*x_kal;
     Pm = H*P*H' +R;
     K = P*H'*inv(Pm);       
     x_kal = x_kal + K*(y-ym);
     P = P - K*H*P;

== matlab function KF_R_estimation/Voltage_estimator/Kalman Filtering Step1 ==
  data: w0 input; Ad output; Ts input
function Ad = A_d(w0,Ts)
Ad =[cos(w0*Ts),sin(w0*Ts)/w0, 0;
    -sin(w0*Ts)*w0,cos(w0*Ts),0;
    0,0,1];

== matlab function KF_R_estimation/Subsystem/Kalman Filtering Step ==
  data: y input; A input; Q input; R input; x input; H input; x_kal output; P_old input; P output
function [x_kal, P] = kalman_filter(y, A, Q, R, x, H, P_old)

== matlab function KF_R_estimation/Subsystem1/Subsystem/MATLAB Function4 ==
  data: a_l input; b_l input; c_l input; current input; Tj input; Rds_on output
function Rds_on = estimate_Rds_on(a_l,b_l,c_l,current,Tj)
     I=[1; current; current^2; current^3;current^4;current.^5;current.^6]
     a=  a_l*I*1000 
     b=  b_l*I*1000
     c=  c_l*I*1000
     Rds_on=a+b*Tj+c*Tj^2
        
end

== matlab function KF_R_estimation/Subsystem/Kalman Filtering Step1 ==
  data: w0 input; Ad output; Ts input
function Ad = A_d(w0,Ts)
Ad =[cos(w0*Ts),sin(w0*Ts)/w0,0,0,0,0;
    -sin(w0*Ts)*w0,cos(w0*Ts),0,0,0,0;
    0,0,cos(w0*Ts),sin(w0*Ts)/w0,0,0;
    0,0,-sin(w0*Ts)*w0,cos(w0*Ts),0,0;
    0,0,0,0,1,0;
    0,0,0,0,0,1];

== matlab function KF_R_estimation/Subsystem/Offset_estimator/MATLAB Function ==
  data: offset_before input; offset_after output; y input; k_2 input; k_2 output
function [offset_after,k_2] = offset_estimator(offset_before,y, k_2)

offset_after=(offset_before*(k_2)+y)/(k_2+1)
k_2=k_2+1
